simulink model "phase2_pure_simulink"  (R2026a)
settings: Solver=VariableStepAuto
libraries: simulink x2
settings Model: Creator=User  LastModifiedBy=User

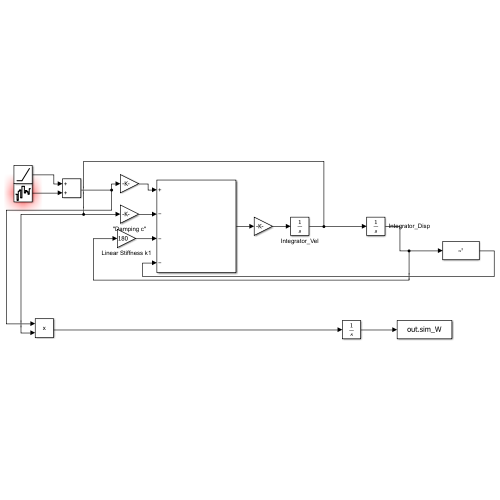
[thumbnail: Simulink's stored preview of the top-level diagram]
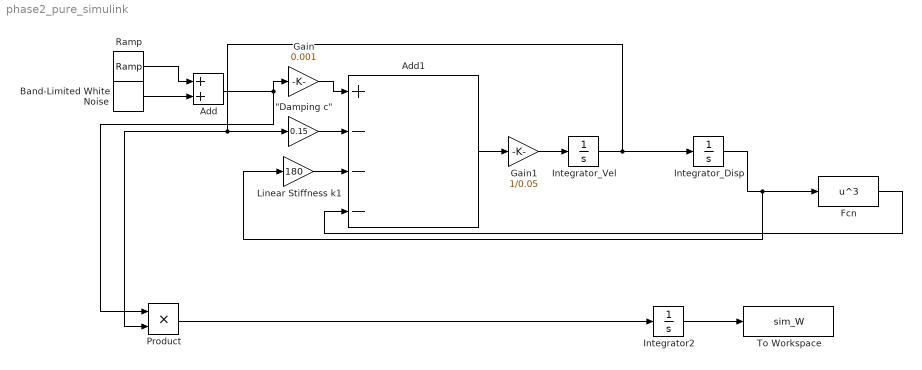
== system phase2_pure_simulink ==
  "\"Damping c\"" : Gain  Gain=0.15
  Add : Sum
  Add1 : Sum  Inputs=+---
  Band-Limited White Noise : simulink/Sources/Band-Limited White Noise  Cov=0.1  Ts=0.1  seed=noise_seed
  Fcn : Fcn  Expr=u^3
  Gain : Gain  Gain=0.001
  Gain1 : Gain  Gain=1/0.05
  Integrator2 : Integrator
  Integrator_Disp : Integrator
  Integrator_Vel : Integrator
  Linear Stiffness k1 : Gain  Gain=180
  Product : Product
  Ramp : simulink/Sources/Ramp  slope=3000  start=0.1  InitialOutput=0
  To Workspace : ToWorkspace  VariableName=sim_W  SampleTime=-1
  wires:
  Integrator_Vel/1 -> Product/2, "\"Damping c\""/1, Integrator_Disp/1
  Band-Limited White Noise/1 -> Add/2
  Add/1 -> Gain/1, Product/1
  Gain/1 -> Add1/1
  Add1/1 -> Gain1/1
  Gain1/1 -> Integrator_Vel/1
  "\"Damping c\""/1 -> Add1/2
  Linear Stiffness k1/1 -> Add1/3
  Integrator_Disp/1 -> Linear Stiffness k1/1, Fcn/1
  Fcn/1 -> Add1/4
  Product/1 -> Integrator2/1
  Integrator2/1 -> To Workspace/1
  Ramp/1 -> Add/1
